simulink model "switches"  (Simulink 7.8)
settings: Solver=ode45  StartTime=0.0  StopTime=0.1  RelTol=1e-3
libraries: simulink x2
settings Model: Creator=yshoukry  LastModifiedBy=yshoukry

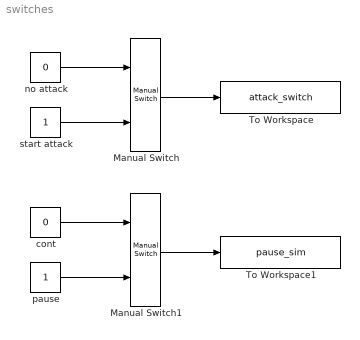
== system switches ==
  Manual Switch : simulink/Signal Routing/Manual Switch  sw=1  action=0  varsize=off
  Manual Switch1 : simulink/Signal Routing/Manual Switch  sw=1  action=0  varsize=off
  To Workspace : ToWorkspace  VariableName=attack_switch  SampleTime=-1  SaveFormat=Array
  To Workspace1 : ToWorkspace  VariableName=pause_sim  SampleTime=-1  SaveFormat=Array
  cont : Constant  Value=0
  no attack : Constant  Value=0
  pause : Constant
  start attack : Constant
  wires:
  Manual Switch/1 -> To Workspace/1
  no attack/1 -> Manual Switch/1
  start attack/1 -> Manual Switch/2
  Manual Switch1/1 -> To Workspace1/1
  cont/1 -> Manual Switch1/1
  pause/1 -> Manual Switch1/2
